simulink model "PID_smithpredictor"  (R2024a)
settings: Solver=FixedStepAuto  StartTime=0.0  StopTime=inf  RelTol=1e-9  EnableMultiTasking=on
values from neighbouring files (symbols this model uses):
  A = 4*3.14*0.02^2    (= 0.005024)    [systemIdentification.m]
  g = 9.81    [systemIdentification.m]
  m = 0.00283    [systemIdentification.m]
  rho = 1.225    [systemIdentification.m]
undefined symbols (not defined in the file or in its folder): alpha, beta, C_D, disturb_magnitude, disturb_time, ln, z_0
libraries: arduinolib x2
settings Model: ExtModeTrigDuration=2  Creator=twallema  LastModifiedBy=twallema
settings SolverCC: AlgebraicLoopSolver=TrustRegion
settings OptimizationCC: EnhancedBackFolding=on  PassReuseOutputArgsThreshold=0  MaxStackSize=64  OptimizeBlockOrder=speed  DifferentSizesBufferReuse=on  OptimizationCustomize=off
settings DebuggingCC: ParameterTunabilityLossMsg=error  UnconnectedInputMsg=warning  UnconnectedOutputMsg=warning  UnconnectedLineMsg=warning
settings HardwareCC: ProdBitPerInt=16  ProdBitPerPointer=16  ProdBitPerSizeT=16  ProdBitPerPtrDiffT=16  ProdLargestAtomicFloat=None  ProdWordSize=8  ProdHWDeviceType=Atmel->AVR  UseEmbeddedCoderFeatures=off  UseSimulinkCoderFeatures=off
settings ModelReferenceCC: EnableRefExpFcnMdlSchedulingChecks=on
settings SFSimCC: MATLABDynamicMemAlloc=off  CustomCodeUndefinedFunction=UseInterfaceOnly
settings RTWCC: Description=Embedded Coder  SystemTargetFile=ert.tlc  HardwareBoard=Arduino Uno  TemplateMakefile=ert_default_tmf  GenerateReport=on  Toolchain=Arduino AVR  BuildConfiguration=Faster Runs  LaunchReport=on  GPUComputeCapability=3.5  DLArmComputeVersion=19.05
settings CodeAppCC: ForceParamTrailComments=on  OperatorAnnotations=on
settings ERTTargetCC: ERTCustomFileBanners=off  SupportContinuousTime=on  SupportNonInlinedSFcns=on  RemoveResetFunc=off  SupportVariableSizeSignals=on  ModelStepFunctionPrototypeControlCompliant=off  ExtModeStaticAllocSize=250

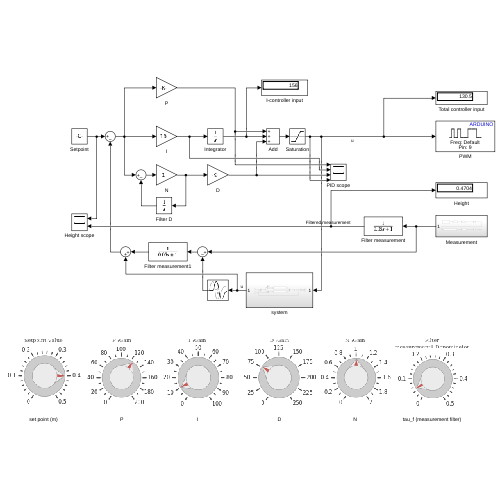
[thumbnail: Simulink's stored preview of the top-level diagram]
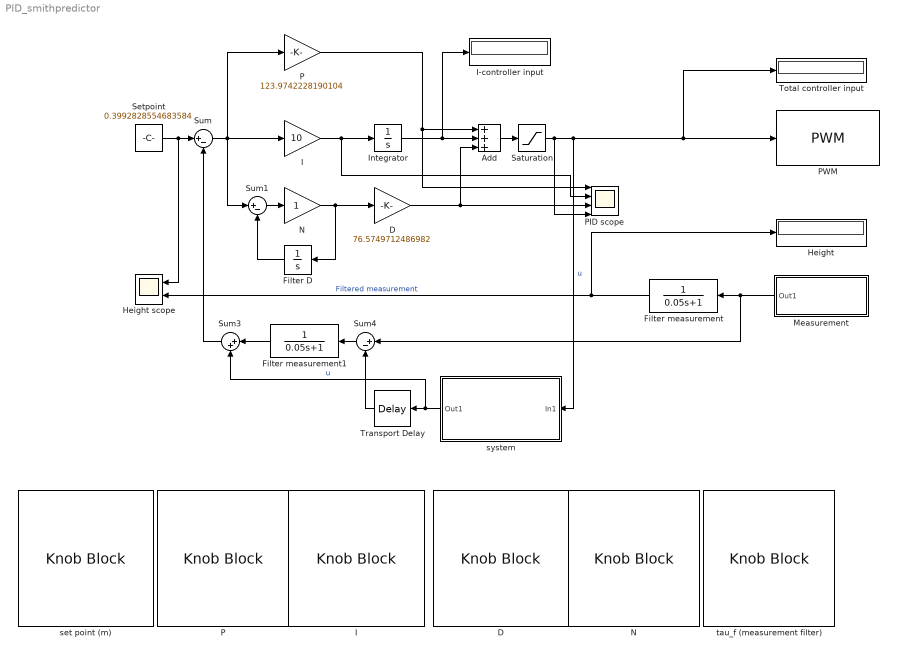
== system PID_smithpredictor ==
  Add : Sum  Inputs=+++
  D : KnobBlock  ScaleMax=250
  "D " : Gain  Gain=76.5749712486982
  Filter D : Integrator
  Filter measurement : TransferFcn  Denominator=[0.05,1]
  Filter measurement1 : TransferFcn  Denominator=[0.05,1]
  Height : Display
  Height scope : Scope  NumInputPorts=2
  I : KnobBlock
  "I " : Gain  Gain=10
  I-controller input : Display
  Integrator : Integrator  InitialCondition=151
  Measurement : Subsystem
  N : KnobBlock  ScaleMax=2
  "N " : Gain
  P : KnobBlock  ScaleMax=200
  "P " : Gain  Gain=123.9742228190104
  PID scope : Scope  NumInputPorts=4
  PWM : arduinolib/PWM  pinNumber=9  frequencyType=Default  desiredFrequency=490.2  achievableFrequency=490.2
  Saturation : Saturate  UpperLimit=255  LowerLimit=0
  Setpoint : Constant  Value=0.3992828554683584
  Sum : Sum  Inputs=|+-
  Sum1 : Sum  Inputs=|+-
  Sum3 : Sum  Inputs=|++
  Sum4 : Sum  Inputs=|+-
  Total controller input : Display
  Transport Delay : TransportDelay  DelayTime=0.5  InitialOutput=z_0(1)
  set point (m) : KnobBlock  ScaleMax=0.50  TickInterval=0.1
  system : Subsystem
  tau_f (measurement filter) : KnobBlock  ScaleMax=0.5  TickInterval=0.1
  wires:
  Setpoint/1 -> Sum/1, Height scope/1
  Sum/1 -> "P "/1, "I "/1, Sum1/1
  Saturation/1 -> system/1(In1), Total controller input/1, PWM/1, PID scope/4  "u"
  Add/1 -> Saturation/1
  "I "/1 -> PID scope/2, Integrator/1
  Integrator/1 -> I-controller input/1, Add/2
  Sum1/1 -> "N "/1
  Filter D/1 -> Sum1/2
  "N "/1 -> Filter D/1, "D "/1
  "D "/1 -> Add/3, PID scope/3
  Filter measurement/1 -> Height scope/2, Height/1  "Filtered measurement"
  "P "/1 -> PID scope/1, Add/1
  system/1(Out1) -> Sum3/2, Transport Delay/1  "u"
  Transport Delay/1 -> Sum4/2
  Sum3/1 -> Sum/2
  Measurement/1(Out1) -> Sum4/1, Filter measurement/1
  Filter measurement1/1 -> Sum3/1
  Sum4/1 -> Filter measurement1/1

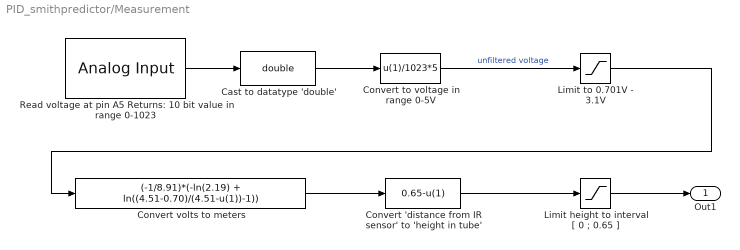
== system PID_smithpredictor/Measurement ==
  Cast to datatype 'double' : DataTypeConversion  OutDataTypeStr=double  SaturateOnIntegerOverflow=off  RndMeth=Floor
  Convert 'distance from IR sensor' to 'height in tube' : Fcn  Expr=0.65-u(1)
  Convert to voltage in range 0-5V : Fcn  Expr=u(1)/1023*5
  Convert volts to meters : Fcn  Expr=(-1/8.91)*(-ln(2.19) + ln((4.51-0.70)/(4.51-u(1))-1))
  Limit height to interval [ 0 ; 0.65 ] : Saturate  UpperLimit=0.65  LowerLimit=0
  Limit to 0.701V - 3.1V : Saturate  UpperLimit=3.1  LowerLimit=0.701
  Read voltage at pin A5 Returns: 10 bit value in range 0-1023 : arduinolib/Analog Input  pinNumber=5  ReadResultsOnly=off  ConversionTriggerSource=Software  ExternalTriggerType=uint32(0)  OutputDataType=uint16  EnableConversionCompleteNotify=off  EnableOuputStatus=off  SampleTime=0.1  blockPlatform=arduino
  Out1 : Outport  VectorParamsAs1DForOutWhenUnconnected=off
  wires:
  Convert 'distance from IR sensor' to 'height in tube'/1 -> Limit height to interval [ 0 ; 0.65 ]/1
  Cast to datatype 'double'/1 -> Convert to voltage in range 0-5V/1
  Read voltage at pin A5 Returns: 10 bit value in range 0-1023/1 -> Cast to datatype 'double'/1
  Limit height to interval [ 0 ; 0.65 ]/1 -> Out1/1
  Convert volts to meters/1 -> Convert 'distance from IR sensor' to 'height in tube'/1
  Limit to 0.701V - 3.1V/1 -> Convert volts to meters/1
  Convert to voltage in range 0-5V/1 -> Limit to 0.701V - 3.1V/1  "unfiltered voltage"

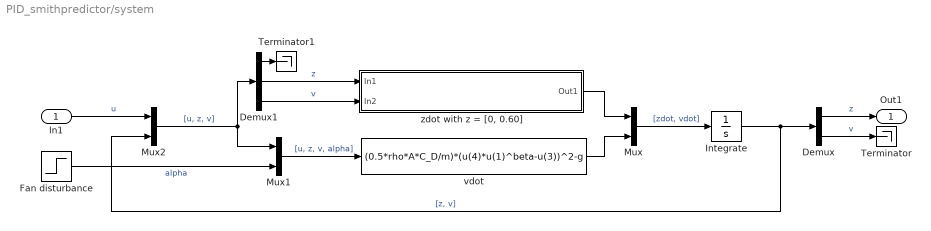
== system PID_smithpredictor/system ==
  In1 : Inport
  Demux : Demux  Outputs=2
  Demux1 : Demux  Outputs=3
  Fan disturbance : Step  Time=disturb_time  Before=alpha  After=alpha*(1+disturb_magnitude/100)  SampleTime=0
  Integrate : Integrator  InitialCondition=z_0
  Mux : Mux  Inputs=2
  Mux1 : Mux  Inputs=2
  Mux2 : Mux  Inputs=2
  Terminator : Terminator
  Terminator1 : Terminator
  vdot : Fcn  Expr=(0.5*rho*A*C_D/m)*(u(4)*u(1)^beta-u(3))^2-g
  "zdot with z = [0, 0.60]" : Subsystem
  Out1 : Outport  VectorParamsAs1DForOutWhenUnconnected=off
  wires:
  vdot/1 -> Mux/2
  Mux2/1 -> Mux1/1, Demux1/1  "[u, z, v]"
  In1/1 -> Mux2/1  "u"
  Integrate/1 -> Demux/1, Mux2/2  "[z, v]"
  Mux/1 -> Integrate/1  "[zdot, vdot]"
  Demux1/1 -> Terminator1/1
  Demux1/3 -> "zdot with z = [0, 0.60]"/2(In2)  "v"
  Demux1/2 -> "zdot with z = [0, 0.60]"/1(In1)  "z"
  "zdot with z = [0, 0.60]"/1(Out1) -> Mux/1
  Mux1/1 -> vdot/1  "[u, z, v, alpha]"
  Fan disturbance/1 -> Mux1/2  "alpha"
  Demux/1 -> Out1/1  "z"
  Demux/2 -> Terminator/1  "v"

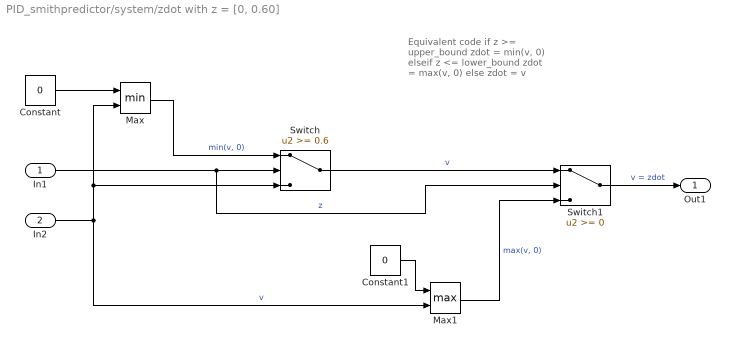
== system PID_smithpredictor/system/zdot with z = [0, 0.60] ==
  note: Equivalent code
      |
      | if z >= upper_bound
      | zdot = min(v, 0)
      | elseif z <= lower_bound
      | zdot = max(v, 0)
      | else
      | zdot = v
  In1 : Inport
  In2 : Inport  Port=2
  Constant : Constant  Value=0
  Constant1 : Constant  Value=0
  Max : MinMax  Inputs=2
  Max1 : MinMax  Function=max  Inputs=2
  Switch : Switch  Threshold=0.6  SaturateOnIntegerOverflow=off  InputSameDT=off
  Switch1 : Switch  SaturateOnIntegerOverflow=off  InputSameDT=off
  Out1 : Outport
  wires:
  Max1/1 -> Switch1/3  "max(v, 0)"
  Constant/1 -> Max/1
  Constant1/1 -> Max1/1
  Switch/1 -> Switch1/1  "v"
  Max/1 -> Switch/1  "min(v, 0)"
  Switch1/1 -> Out1/1  "v = zdot"
  In1/1 -> Switch/2, Switch1/2  "z"
  In2/1 -> Max/2, Switch/3, Max1/2  "v"
